simulink model "exp1_4_a"  (R2014a)
settings: Solver=FixedStepDiscrete  StartTime=0.0  StopTime=inf  RelTol=1e-3
libraries: xpcdiamondlib x2, slrtlib x2
settings Model: BufferReuse=off  Creator=jyang168  LastModifiedBy=ywang744
settings SolverCC: EnableConcurrentExecution=on
settings OptimizationCC: BlockReduction=off  OptimizeBlockIOStorage=off  BufferReuse=off  GlobalBufferReuse=off  ExpressionFolding=off  LocalBlockOutputs=off
settings HardwareCC: ProdIntDivRoundTo=Zero  ProdEndianess=LittleEndian  ProdHWDeviceType=Generic->32-bit x86 compatible
settings RTWCC: SystemTargetFile=slrt.tlc  TemplateMakefile=slrt_default_tmf  Description=Simulink Real-Time  ProcessScript=slrt_make_rtw_hook  RTWCompilerOptimization=On
settings SimulinkRealTimeCC: GeneratePreprocessorConditionals=Disable all  EnableShiftOperators=on  xPCisDownloadable=off

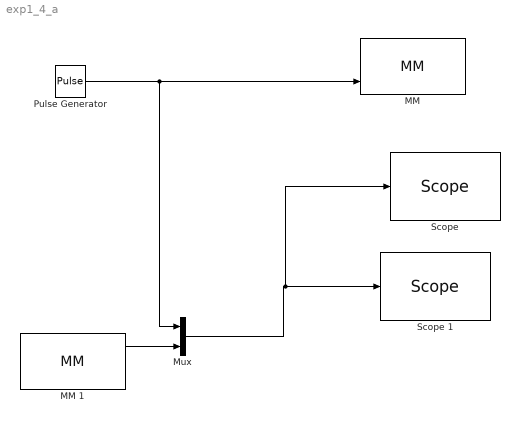
== system exp1_4_a ==
  "MM " : xpcdiamondlib/D//A/MM   channel=[1,2]  range=[5]  reset=[1]  initValue=[0]  sampleTime=0.1  base=0x300
  MM 1 : xpcdiamondlib/A//D/MM   numChans=2  range=-5V to 5V  coupling=16 single-ended channels  showStatus=off  sampleTime=0.1  base=0x300
  Mux : Mux  Inputs=2
  Pulse Generator : DiscretePulseGenerator  Period=20  PulseWidth=10  SampleTime=0.1
  "Scope " : slrtlib/Displays and Logging/Scope   scopeno=1  scopetype=Target  autostart=on  viewmode=Graphical sliding  formatstr='%15.6f'  grid=on  ylimits=[0,0]  nosamples=250  noprepostsamples=0  interleave=1  triggermode=FreeRun  triggersignal=1  trigsignalfromport=off  triggerlevel=0.0  triggerslope=Either  triggerscope=1  triggersample=0  filename=data.dat  mode=Lazy  writesize=512  autorestart=off  dynamicfilemode=off  maxwritefilesize=512*1024^2
  Scope 1 : slrtlib/Displays and Logging/Scope   scopeno=2  scopetype=Target  autostart=on  viewmode=Numerical  formatstr='%15.6f'  grid=on  ylimits=[0,0]  nosamples=250  noprepostsamples=0  interleave=1  triggermode=FreeRun  triggersignal=1  trigsignalfromport=off  triggerlevel=0.0  triggerslope=Either  triggerscope=1  triggersample=0  filename=data.dat  mode=Lazy  writesize=512  autorestart=off  dynamicfilemode=off  maxwritefilesize=512*1024^2
  wires:
  Pulse Generator/1 -> "MM "/2, Mux/1
  MM 1/1 -> Mux/2
  Mux/1 -> "Scope "/1, Scope 1/1
